simulink model "simulink_project_sinusoidal"  (R2021a)
settings: Solver=VariableStepAuto  StartTime=0.0  StopTime=10.0  RelTol=1e-3
values from neighbouring files (symbols this model uses):
  c1 = 100    [ode.m]
  c2 = 1000    [ode.m]
  k1 = 1e4    (= 10000)    [ode.m]
  k2 = 1e5    (= 100000)    [ode.m]
  m1 = 10    [ode.m]
  m2 = 100    [ode.m]
settings Model: Creator=eshannayak  LastModifiedBy=eshannayak

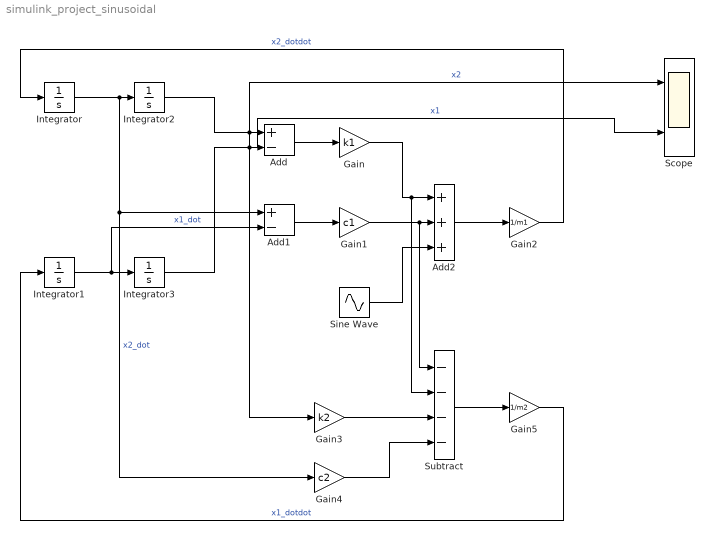
== system simulink_project_sinusoidal ==
  Add : Sum  Inputs=+-
  Add1 : Sum  Inputs=+-
  Add2 : Sum  Inputs=+++
  Gain : Gain  Gain=k1
  Gain1 : Gain  Gain=c1
  Gain2 : Gain  Gain=1/m1
  Gain3 : Gain  Gain=k2
  Gain4 : Gain  Gain=c2
  Gain5 : Gain  Gain=1/m2
  Integrator{,1..3} (4 alike) : Integrator
  Scope : Scope  NumInputPorts=2
  Sine Wave : Sin  Amplitude=3  Frequency=10  SampleTime=0
  Subtract : Sum  Inputs=----
  wires:
  Gain2/1 -> Integrator/1  "x2_dotdot"
  Integrator/1 -> Add1/1, Gain4/1, Integrator2/1  "x2_dot"
  Gain5/1 -> Integrator1/1  "x1_dotdot"
  Integrator1/1 -> Add1/2, Integrator3/1  "x1_dot"
  Integrator2/1 -> Gain3/1, Add/1, Scope/1  "x2"
  Integrator3/1 -> Scope/2, Add/2  "x1"
  Add/1 -> Gain/1
  Add1/1 -> Gain1/1
  Sine Wave/1 -> Add2/3
  Gain1/1 -> Subtract/1, Add2/2
  Gain/1 -> Subtract/2, Add2/1
  Add2/1 -> Gain2/1
  Gain3/1 -> Subtract/3
  Gain4/1 -> Subtract/4
  Subtract/1 -> Gain5/1
